simulink model "Truck_ACC_Project"  (R2026a)
settings: Solver=ode4  FixedStep=0.01
settings Model: Creator=adhav  LastModifiedBy=adhav

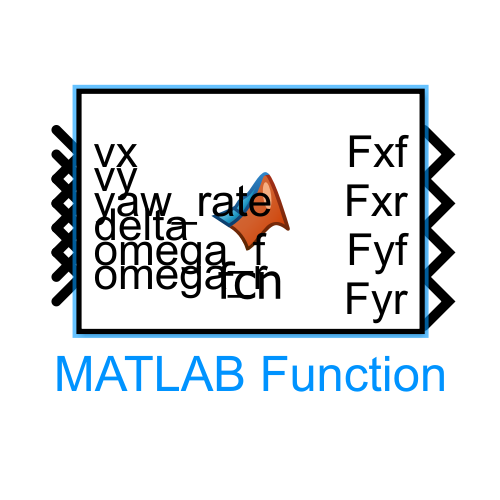
[thumbnail: Simulink's stored preview of the top-level diagram]
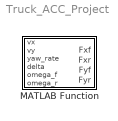
== system Truck_ACC_Project ==
  MATLAB Function : MATLAB Function  TreatAsAtomicUnit=on

== matlab function Truck_ACC_Project/MATLAB Function ==
  data: vx input; Fxf output; vy input; yaw_rate input; delta input; omega_f input; omega_r input; Fxr output; Fyf output; Fyr output
function [Fxf, Fxr, Fyf, Fyr] = Tire_Forces(vx, vy, yaw_rate, delta, omega_f, omega_r)
% MAGIC FORMULA TIRE MODEL
% Translates Equations 32 and 33 from the IEEE paper using Tables III & IV.

    %% 1. Define Parameters (From Table IV)
    a = 3.5;      % Front wheel to center of mass distance (m)
    b = 1.5;      % Rear wheel to center of mass distance (m)
    Re = 0.51;    % Wheel rolling radius (m)
    
    %% 2. Define Tire Parameters (From Table III)
    % Longitudinal Forces (Fxf, Fxr)
    B_kf = 8.61;  C_kf = 1.58;  D_kf = 22053;  E_kf = 0.5624;
    B_kr = 8.61;  C_kr = 1.58;  D_kr = 44625;  E_kr = 0.5624;
    
    % Lateral Forces (Fyf, Fyr)
    B_af = 6.59;  C_af = 2.42;  D_af = 22053;  E_af = -0.3028;
    B_ar = 6.59;  C_ar = 2.42;  D_ar = 44625;  E_ar = -0.3028;
    
    %% 3. Unit Conversions
    % delta is constrained to [-10, 10] degrees in the paper, convert to radians
    delta_rad = deg2rad(delta); 
    
    % Safety buffer to prevent division by zero
    epsilon = 1e-6; 

    %% 4. Calculate Slip Ratios (Equation 32)
    kf = (omega_f * Re - vx) / max(omega_f * Re, vx + epsilon);
    kr = (omega_r * Re - vx) / max(omega_r * Re, vx + epsilon);

    %% 5. Calculate Slip Angles (Equation 33)
    % Determine tire longitudinal and lateral velocities
    v_alpha_f = vx * cos(delta_rad) + (vy + a * yaw_rate) * sin(delta_rad);
    v_beta_f  = (vy + a * yaw_rate) * cos(delta_rad) - vx * sin(delta_rad);
    
    v_alpha_r = vx;
    v_beta_r  = vy - b * yaw_rate;
    
    % Calculate slip angles
    alpha_f = sign(v_alpha_f) * atan(v_beta_f / (abs(v_alpha_f) + epsilon));
    alpha_r = sign(v_alpha_r) * atan(v_beta_r / (abs(v_alpha_r) + epsilon));

    %% 6. Magic Formula Equation (Bottom of Section IV-A)
    % Front Longitudinal Force (Fxf)
    Fxf = D_kf * sin(C_kf * atan(B_kf * kf - E_kf * (B_kf * kf - atan(B_kf * kf))));
    
    % Rear Longitudinal Force (Fxr)
    Fxr = D_kr * sin(C_kr * atan(B_kr * kr - E_kr * (B_kr * kr - atan(B_kr * kr))));
    
    % Front Lateral Force (Fyf)
    Fyf = D_af * sin(C_af * atan(B_af * alpha_f - E_af * (B_af * alpha_f - atan(B_af * alpha_f))));
    
    % Rear Lateral Force (Fyr)
    Fyr = D_ar * sin(C_ar * atan(B_ar * alpha_r - E_ar * (B_ar * alpha_r - atan(B_ar * alpha_r))));
end
